simulink model "input_signal_test"  (Simulink 7.4)
settings: Solver=VariableStepDiscrete  StartTime=0.0  StopTime=10.0  MaxStep=0.01  RelTol=1e-3
values from neighbouring files (symbols this model uses):
  da = struct('coefficient', 8.5*10^(-3)          , 'maxError', 25*10^(-3)          , 'actualError', -1000          , 'type', 1          , 'frequency', 0          , 'order', 0          , 'tf', 1          , 'on', 1          )    [a2_data_input_examsim1.m]
  dp = struct('coefficient', 6*10^(-2)          , 'maxError', 6*10^(-4)          , 'actualError', -1000          , 'type', 2          , 'frequency', 10          , 'order', -10          , 'tf', Gd          , 'on', 1          )    [a2_data_input_examsim1.m]
  ds = struct('coefficient', 1*10^(-3)          , 'maxError', 1*10^(-4)          , 'actualError', -1000          , 'type', 2          , 'frequency', 10000          , 'order', -10          , 'tf', 1          , 'on', 1          )    [a2_data_input_examsim1.m]
  r = struct('coefficient', 1          , 'maxError', 1.5*10^(-1)          , 'actualError', -1000          , 'type', 1          , 'frequency', 0          , 'order', 0          , 'tf', Gr          , 'on', 1          )    [a2_data_input_examsim1.m]
libraries: cstblocks x4
settings Model: Creator=Vittorio  LastModifiedBy=Vittorio

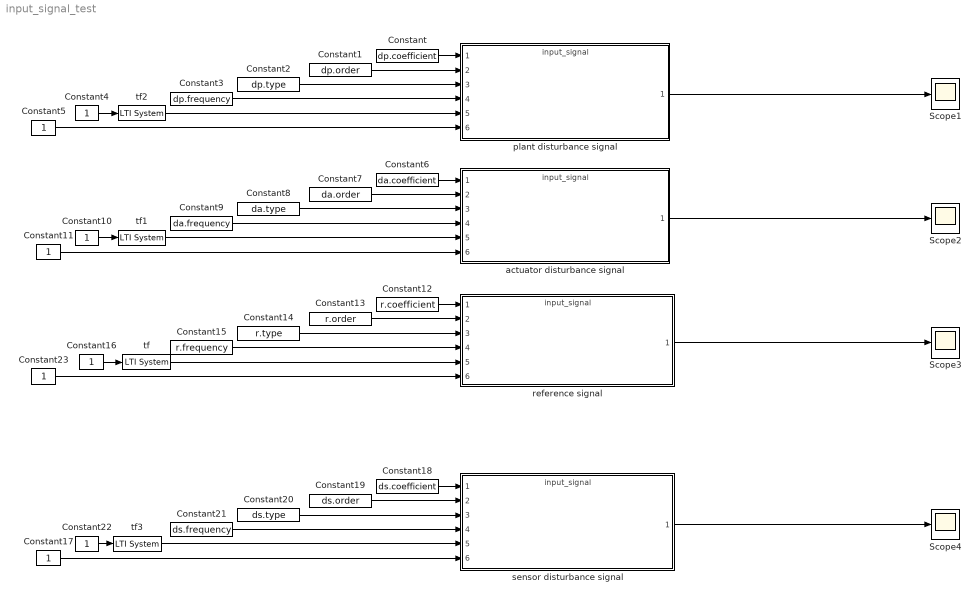
== system input_signal_test ==
  Constant : Constant  Value=dp.coefficient  OutDataType=fixdt(1, 16)  OutScaling=2^0
  Constant1 : Constant  Value=dp.order  OutDataType=fixdt(1, 16)  OutScaling=2^0
  Constant{4..5,10..11,16..17,22..23} (8 alike) : Constant  OutDataType=fixdt(1, 16)  OutScaling=2^0
  Constant12 : Constant  Value=r.coefficient  OutDataType=fixdt(1, 16)  OutScaling=2^0
  Constant13 : Constant  Value=r.order  OutDataType=fixdt(1, 16)  OutScaling=2^0
  Constant14 : Constant  Value=r.type  OutDataType=fixdt(1, 16)  OutScaling=2^0
  Constant15 : Constant  Value=r.frequency  OutDataType=fixdt(1, 16)  OutScaling=2^0
  Constant18 : Constant  Value=ds.coefficient  OutDataType=fixdt(1, 16)  OutScaling=2^0
  Constant19 : Constant  Value=ds.order  OutDataType=fixdt(1, 16)  OutScaling=2^0
  Constant2 : Constant  Value=dp.type  OutDataType=fixdt(1, 16)  OutScaling=2^0
  Constant20 : Constant  Value=ds.type  OutDataType=fixdt(1, 16)  OutScaling=2^0
  Constant21 : Constant  Value=ds.frequency  OutDataType=fixdt(1, 16)  OutScaling=2^0
  Constant3 : Constant  Value=dp.frequency  OutDataType=fixdt(1, 16)  OutScaling=2^0
  Constant6 : Constant  Value=da.coefficient  OutDataType=fixdt(1, 16)  OutScaling=2^0
  Constant7 : Constant  Value=da.order  OutDataType=fixdt(1, 16)  OutScaling=2^0
  Constant8 : Constant  Value=da.type  OutDataType=fixdt(1, 16)  OutScaling=2^0
  Constant9 : Constant  Value=da.frequency  OutDataType=fixdt(1, 16)  OutScaling=2^0
  Scope{1..4} (4 alike) : Scope
      Scope3 settings: SaveName=ScopeData2
      Scope4 settings: SaveName=ScopeData3
  actuator disturbance signal : ModelReference  ModelNameDialog=input_signal  SimulationMode=Accelerator  ModelReferenceVersion=1.13  CopyOfModelName=input_signal
  plant disturbance signal : ModelReference  ModelNameDialog=input_signal  SimulationMode=Accelerator  ModelReferenceVersion=1.13  CopyOfModelName=input_signal
  reference signal : ModelReference  ModelNameDialog=input_signal  SimulationMode=Accelerator  ModelReferenceVersion=1.13  CopyOfModelName=input_signal
  sensor disturbance signal : ModelReference  ModelNameDialog=input_signal  SimulationMode=Accelerator  ModelReferenceVersion=1.13  CopyOfModelName=input_signal
  tf : cstblocks/LTI System  SystemSampleTime=-1  sys=r.tf  IC=[]
  tf1 : cstblocks/LTI System  SystemSampleTime=-1  sys=da.tf  IC=[]
  tf2 : cstblocks/LTI System  SystemSampleTime=-1  sys=dp.tf  IC=[]
  tf3 : cstblocks/LTI System  SystemSampleTime=-1  sys=ds.tf  IC=[]
  wires:
  Constant/1 -> plant disturbance signal/1
  Constant1/1 -> plant disturbance signal/2
  Constant2/1 -> plant disturbance signal/3
  Constant3/1 -> plant disturbance signal/4
  tf2/1 -> plant disturbance signal/5
  Constant6/1 -> actuator disturbance signal/1
  Constant7/1 -> actuator disturbance signal/2
  Constant8/1 -> actuator disturbance signal/3
  Constant9/1 -> actuator disturbance signal/4
  tf1/1 -> actuator disturbance signal/5
  Constant11/1 -> actuator disturbance signal/6
  Constant12/1 -> reference signal/1
  Constant13/1 -> reference signal/2
  Constant14/1 -> reference signal/3
  Constant15/1 -> reference signal/4
  tf/1 -> reference signal/5
  Constant23/1 -> reference signal/6
  Constant18/1 -> sensor disturbance signal/1
  Constant19/1 -> sensor disturbance signal/2
  Constant20/1 -> sensor disturbance signal/3
  Constant21/1 -> sensor disturbance signal/4
  tf3/1 -> sensor disturbance signal/5
  Constant17/1 -> sensor disturbance signal/6
  Constant16/1 -> tf/1
  Constant10/1 -> tf1/1
  Constant4/1 -> tf2/1
  Constant22/1 -> tf3/1
  Constant5/1 -> plant disturbance signal/6
  plant disturbance signal/1 -> Scope1/1
  actuator disturbance signal/1 -> Scope2/1
  reference signal/1 -> Scope3/1
  sensor disturbance signal/1 -> Scope4/1
